simulink model "assignment_11_adaptive_final"  (R2022b)
settings: Solver=VariableStepAuto  StartTime=0.0  StopTime=30  RelTol=1e-3
values from neighbouring files (symbols this model uses):
  dq0 = [0;0;0]    [assignment_10.m]    (also in assignment_11.m; assignment_12.m; assignment_13.m; assignment_6.m)
  K_env = 1000    [assignment_11.m]    (also in assignment_12.m = 100; assignment_13.m = 100)
  Kd = 100    [assignment_10.m]    (also in assignment_11.m = 1000; assignment_12.m; assignment_6.m = 1000; assignment_7.m = diag(2 * xi .* w))
  Kp = 1000    [assignment_10.m]    (also in assignment_11.m = 10000; assignment_12.m; assignment_6.m; assignment_7.m = diag(w .* w))
  q0 = [0;0;0]    [assignment_10.m]    (also in assignment_11.m; assignment_12.m; assignment_13.m = [0; pi/2; -pi/2]; assignment_6.m)
  x_desired = direct_kinematics(q_desired)    [assignment_11.m]
  x_rest_env = direct_kinematics(q_rest_env)    [assignment_11.m]    (also in assignment_12.m; assignment_13.m = x_rest_env(1:3, 1))
settings Model: Creator=acesi  LastModifiedBy=Manu

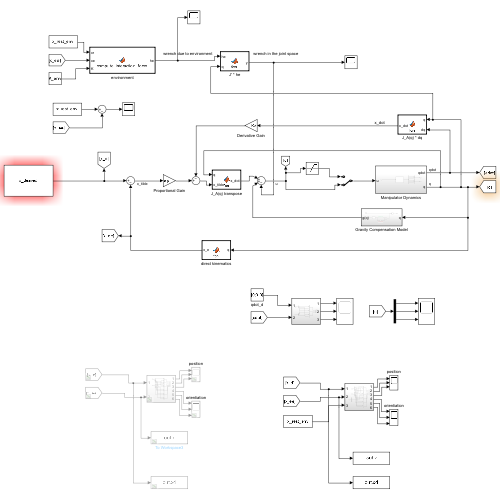
[thumbnail: Simulink's stored preview of the top-level diagram]
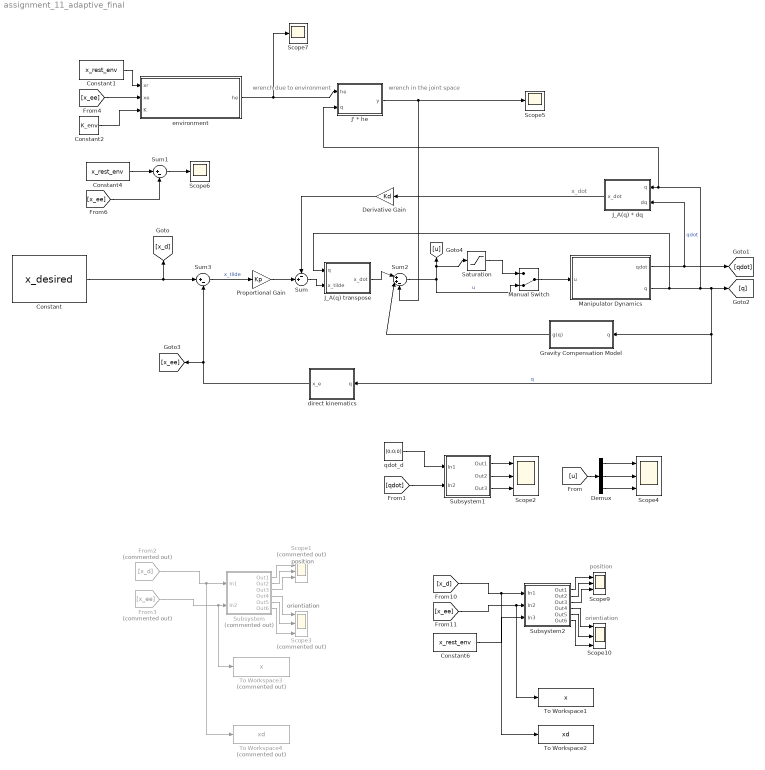
== system assignment_11_adaptive_final ==
  note: wrench in the joint space
  note: wrench due to environment
  note: orientiation
  note: position
  note: x_dot
  note: orientiation
  note: position
  Constant : Constant  Value=x_desired
  Constant1 : Constant  Value=x_rest_env
  Constant2 : Constant  Value=K_env
  Constant4 : Constant  Value=x_rest_env
  Constant6 : Constant  Value=x_rest_env
  Demux : Demux  Outputs=3
  Derivative Gain : Gain  Gain=Kd
  From2 : From  Commented=on  GotoTag=x_d
  From3 : From  Commented=on  GotoTag=x_ee
  Gravity Compensation Model : Subsystem
  J' * he : MATLAB Function  TreatAsAtomicUnit=on
  J_A(q) * dq : MATLAB Function  TreatAsAtomicUnit=on
  J_A(q) transpose : MATLAB Function  TreatAsAtomicUnit=on
  Manipulator Dynamics : Subsystem
  Manual Switch : ManualSwitch  CurrentSetting=0
  Proportional Gain : Gain  Gain=Kp
  Saturation : Saturate  UpperLimit=1000  LowerLimit=-1000
  Scope1 : Scope  Commented=on  NumInputPorts=3
  Scope{2,4,9..10} (4 alike) : Scope  NumInputPorts=3
  Scope3 : Scope  Commented=on  NumInputPorts=3
  Scope5 : Scope
  Scope6 : Scope
  Scope7 : Scope
  Subsystem : Subsystem  Commented=on
  Subsystem1 : Subsystem
  Subsystem2 : Subsystem
  Sum : Sum  Inputs=-+|
  Sum1 : Sum  Inputs=|+-
  Sum2 : Sum  Inputs=|++-
  Sum3 : Sum  Inputs=|+-
  To Workspace1 : ToWorkspace  VariableName=x  SaveFormat=Timeseries  SampleTime=-1
  To Workspace2 : ToWorkspace  VariableName=xd  SaveFormat=Timeseries  SampleTime=-1
  To Workspace3 : ToWorkspace  Commented=on  VariableName=x  SaveFormat=Timeseries  SampleTime=-1
  To Workspace4 : ToWorkspace  Commented=on  VariableName=xd  SaveFormat=Timeseries  SampleTime=-1
  direct kinematics : MATLAB Function  TreatAsAtomicUnit=on
  environment : MATLAB Function  TreatAsAtomicUnit=on
  qdot_d : Constant  Value=[0;0;0]
  wires:
  Proportional Gain/1 -> Sum/2
  Derivative Gain/1 -> Sum/1
  Manipulator Dynamics/1(qdot) -> J_A(q) * dq/2(dq), [qdot]  "qdot"
  Manipulator Dynamics/2(q) -> J_A(q) transpose/1(q), [q], Gravity Compensation Model/1(q), direct kinematics/1(q), J' * he/2(q), J_A(q) * dq/1(q)  "q"
  Sum2/1 -> [u], Saturation/1, Manual Switch/2  "u"
  Gravity Compensation Model/1(g(q)) -> Sum2/2
  From2/1 -> Subsystem/1(In1), To Workspace4/1
  From3/1 -> To Workspace3/1, Subsystem/2(In2)
  Subsystem/1(Out1) -> Scope1/1
  Subsystem/2(Out2) -> Scope1/2
  Subsystem/3(Out3) -> Scope1/3
  qdot_d/1 -> Subsystem1/1(In1)
  [qdot] -> Subsystem1/2(In2)
  Subsystem1/1(Out1) -> Scope2/1
  Subsystem1/2(Out2) -> Scope2/2
  Subsystem1/3(Out3) -> Scope2/3
  Sum3/1 -> Proportional Gain/1  "x_tilde"
  direct kinematics/1(x_e) -> Sum3/2, [x_ee]
  J_A(q) * dq/1(x_dot) -> Derivative Gain/1
  Sum/1 -> J_A(q) transpose/2(x_tilde)
  J_A(q) transpose/1(x_dot) -> Sum2/1
  Constant/1 -> [x_d], Sum3/1
  Subsystem/4(Out4) -> Scope3/1
  Subsystem/5(Out5) -> Scope3/2
  Subsystem/6(Out6) -> Scope3/3
  Demux/1 -> Scope4/1
  Demux/2 -> Scope4/2
  Demux/3 -> Scope4/3
  [u] -> Demux/1
  Manual Switch/1 -> Manipulator Dynamics/1(u)
  Saturation/1 -> Manual Switch/1
  [x_ee] -> environment/2(xe)
  Constant1/1 -> environment/1(xr)
  Constant2/1 -> environment/3(K)
  environment/1(he) -> J' * he/1(he), Scope7/1
  J' * he/1(y) -> Scope5/1, Sum2/3
  Constant4/1 -> Sum1/1
  [x_ee] -> Sum1/2
  Sum1/1 -> Scope6/1
  Constant6/1 -> Subsystem2/3(In3)
  [x_ee] -> To Workspace1/1, Subsystem2/2(In2)
  Subsystem2/5(Out5) -> Scope10/2
  [x_d] -> Subsystem2/1(In1), To Workspace2/1
  Subsystem2/2(Out2) -> Scope9/2
  Subsystem2/1(Out1) -> Scope9/1
  Subsystem2/3(Out3) -> Scope9/3
  Subsystem2/4(Out4) -> Scope10/1
  Subsystem2/6(Out6) -> Scope10/3

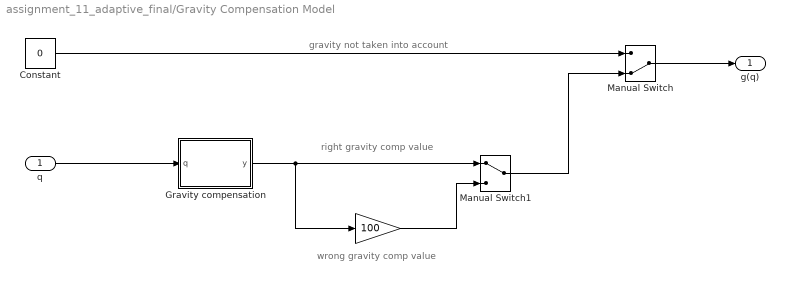
== system assignment_11_adaptive_final/Gravity Compensation Model ==
  note: wrong gravity comp value
  note: right gravity comp value
  note: gravity not taken into account
  q : Inport
  " " : Gain  Gain=100
  Constant : Constant  Value=0
  Gravity compensation : MATLAB Function  TreatAsAtomicUnit=on
  Manual Switch : ManualSwitch  CurrentSetting=0
  Manual Switch1 : ManualSwitch
  g(q) : Outport
  wires:
  Constant/1 -> Manual Switch/1
  Manual Switch/1 -> g(q)/1
  Gravity compensation/1(y) -> " "/1, Manual Switch1/1
  Manual Switch1/1 -> Manual Switch/2
  " "/1 -> Manual Switch1/2
  q/1 -> Gravity compensation/1(q)

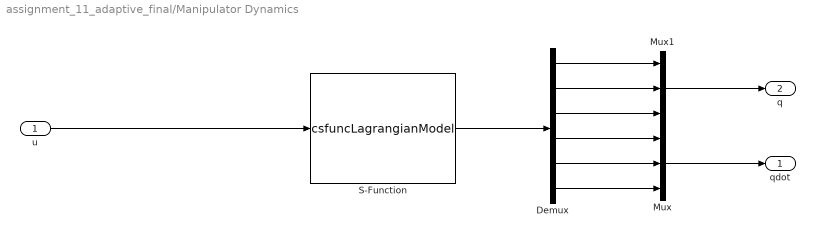
== system assignment_11_adaptive_final/Manipulator Dynamics ==
  u : Inport
  Demux : Demux  Outputs=6
  Mux : Mux  Inputs=3
  Mux1 : Mux  Inputs=3
  S-Function : S-Function  FunctionName=csfuncLagrangianModel  Parameters=q0 dq0  SFunctionDeploymentMode=off  EnableBusSupport=off
  qdot : Outport
  q : Outport  Port=2
  wires:
  u/1 -> S-Function/1
  S-Function/1 -> Demux/1
  Mux1/1 -> q/1
  Mux/1 -> qdot/1
  Demux/6 -> Mux/3
  Demux/5 -> Mux/2
  Demux/4 -> Mux/1
  Demux/3 -> Mux1/3
  Demux/2 -> Mux1/2
  Demux/1 -> Mux1/1

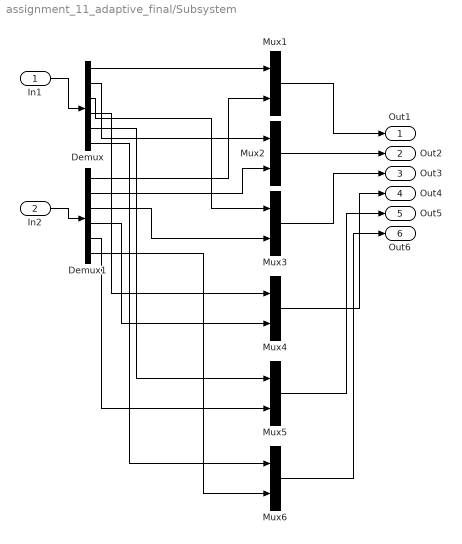
== system assignment_11_adaptive_final/Subsystem ==
  In1 : Inport
  In2 : Inport  Port=2
  Demux : Demux  Outputs=6
  Demux1 : Demux  Outputs=6
  Mux{1..6} (6 alike) : Mux  Inputs=2
  Out1 : Outport
  Out2 : Outport  Port=2
  Out3 : Outport  Port=3
  Out4 : Outport  Port=4
  Out5 : Outport  Port=5
  Out6 : Outport  Port=6
  wires:
  Demux/1 -> Mux1/1
  Demux/3 -> Mux3/1
  Demux/2 -> Mux2/1
  Demux1/1 -> Mux1/2
  Mux2/1 -> Out2/1
  Demux1/3 -> Mux3/2
  Demux1/2 -> Mux2/2
  Mux3/1 -> Out3/1
  Mux1/1 -> Out1/1
  In2/1 -> Demux1/1
  In1/1 -> Demux/1
  Demux1/4 -> Mux4/2
  Demux/4 -> Mux4/1
  Demux/5 -> Mux5/1
  Demux1/5 -> Mux5/2
  Demux/6 -> Mux6/1
  Demux1/6 -> Mux6/2
  Mux4/1 -> Out4/1
  Mux5/1 -> Out5/1
  Mux6/1 -> Out6/1

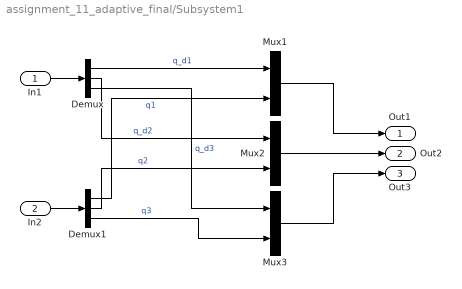
== system assignment_11_adaptive_final/Subsystem1 ==
  In1 : Inport
  In2 : Inport  Port=2
  Demux : Demux  Outputs=3
  Demux1 : Demux  Outputs=3
  Mux1 : Mux  Inputs=2
  Mux2 : Mux  Inputs=2
  Mux3 : Mux  Inputs=2
  Out1 : Outport
  Out2 : Outport  Port=2
  Out3 : Outport  Port=3
  wires:
  Demux/1 -> Mux1/1  "q_d1"
  Demux/3 -> Mux3/1  "q_d3"
  Demux/2 -> Mux2/1  "q_d2"
  Demux1/1 -> Mux1/2  "q1"
  Mux2/1 -> Out2/1
  Demux1/3 -> Mux3/2  "q3"
  Demux1/2 -> Mux2/2  "q2"
  Mux3/1 -> Out3/1
  Mux1/1 -> Out1/1
  In2/1 -> Demux1/1
  In1/1 -> Demux/1

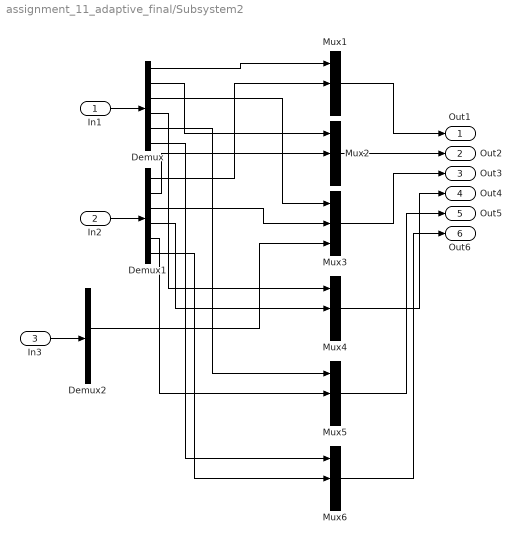
== system assignment_11_adaptive_final/Subsystem2 ==
  In1 : Inport
  In2 : Inport  Port=2
  In3 : Inport  Port=3
  Demux : Demux  Outputs=6
  Demux1 : Demux  Outputs=6
  Demux2 : Demux  Outputs=6
  Mux{1..6} (6 alike) : Mux  Inputs=3
  Out1 : Outport
  Out2 : Outport  Port=2
  Out3 : Outport  Port=3
  Out4 : Outport  Port=4
  Out5 : Outport  Port=5
  Out6 : Outport  Port=6
  wires:
  Demux/1 -> Mux1/1
  Demux/3 -> Mux3/1
  Demux/2 -> Mux2/1
  Demux1/1 -> Mux1/2
  Mux2/1 -> Out2/1
  Demux1/3 -> Mux3/2
  Demux1/2 -> Mux2/2
  Mux3/1 -> Out3/1
  Mux1/1 -> Out1/1
  In2/1 -> Demux1/1
  In1/1 -> Demux/1
  Demux1/4 -> Mux4/2
  Demux/4 -> Mux4/1
  Demux/5 -> Mux5/1
  Demux1/5 -> Mux5/2
  Demux/6 -> Mux6/1
  Demux1/6 -> Mux6/2
  Mux4/1 -> Out4/1
  Mux5/1 -> Out5/1
  Mux6/1 -> Out6/1
  In3/1 -> Demux2/1
  Demux2/3 -> Mux3/3

== matlab function assignment_11_adaptive_final/Gravity Compensation Model/Gravity compensation ==
  data: q input; y output
function y = g(q)

    y = get_G_hardcoded(q);

end

== matlab function assignment_11_adaptive_final/J_A(q) * dq ==
  data: q input; x_dot output; dq input
function x_dot = fcn(q, dq)
    x_dot = get_JA(q) * dq;
end

== matlab function assignment_11_adaptive_final/J_A(q) transpose ==
  data: q input; x_dot output; x_tilde input
function x_dot = fcn(q, x_tilde)
    x_dot = get_JA(q)' * x_tilde;
end

== matlab function assignment_11_adaptive_final/environment ==
  data: xr input; he output; xe input; K input
function he = compute_interaction_force(xr, xe, K)
% xr: rest position of the environment (expressed in the operational space)
% xe: current position of the end effector (expressed in the operational space)
% K: environment spring constant (the env. is modeled as a pure spring)

if xe(3) < xr(3)
    he = zeros(6,1); % no interaction with the environment
else
    % end effector position is larger than the env. rest position
    delta_position = xr - xe;
    he = -K * delta_position; % spring force: f = -kx

    % simulate force only on the z-axis
    he(1:2, 1) = 0; % set x, y components to 0
    he(4:6, 1) = 0; % set orientation components to 0
end

== matlab function assignment_11_adaptive_final/J' * he ==
  data: he input; y output; q input
function y = fcn(he, q)
% maps wrench to joint space (qual'è la nomenclatura corretta?)
y = get_JG(q)' * he;

== matlab function assignment_11_adaptive_final/direct kinematics ==
  data: q input; x_e output
function x_e = fcn(q)
    x_e = direct_kinematics(q);
end
